simulink model "prob1a"  (R2013a)
settings: Solver=ode45  StartTime=0.0  StopTime=12.0  RelTol=1e-3
libraries: powerlib_meascontrol x3
settings Model: Creator=Suddenlink  LastModifiedBy=ngohara

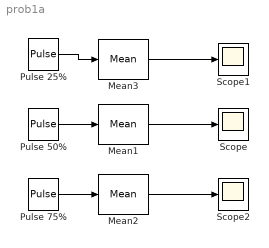
== system prob1a ==
  Mean1 : powerlib_meascontrol/Measurements/Mean  Freq=60  Vinit=0  Ts=0
  Mean2 : powerlib_meascontrol/Measurements/Mean  Freq=60  Vinit=0  Ts=0
  Mean3 : powerlib_meascontrol/Measurements/Mean  Freq=60  Vinit=0  Ts=0
  Pulse 25% : DiscretePulseGenerator  PulseType=Time based  Amplitude=4  Period=4  PulseWidth=25
  Pulse 50% : DiscretePulseGenerator  PulseType=Time based  Amplitude=4  Period=4  PulseWidth=50
  Pulse 75% : DiscretePulseGenerator  PulseType=Time based  Amplitude=4  Period=4  PulseWidth=75
  Scope : Scope
  Scope1 : Scope
  Scope2 : Scope
      settings: SaveName=ScopeData2
  wires:
  Pulse 25%/1 -> Mean3/1
  Pulse 75%/1 -> Mean2/1
  Pulse 50%/1 -> Mean1/1
  Mean1/1 -> Scope/1
  Mean3/1 -> Scope1/1
  Mean2/1 -> Scope2/1
